simulink library "srx_platform"  (Simulink 8.2)
settings: Solver=ode1  StartTime=0.0  StopTime=Inf  FixedStep=0.001  RelTol=1e-3
PostLoadFcn:
  | , if any(exist('dsrtsu_mdlpostloadfcn', 'file') == [2, 3, 6]), try dsrtsu_mdlpostloadfcn('Execute', bdroot); catch fprintf('Error in PostLoadFcn (dsrtsu_mdlpostloadfcn) for model "%s":\n %s\n', bdroot, lasterr); end, end,
libraries: rtican x23, rtiethernetudplib x4, srx_initialize x4, rtiflashlib x2, topr5_adapter x1
(part 1 of 6)
settings Model: DSRTSU_INTERNAL_RTI_VER=450  DSRTSU_INTERNAL_RTI_TYPE=rti1401  DSRTSU_INTERNAL_RTIFPGA=40  Creator=leidos  LastModifiedBy=rushk1

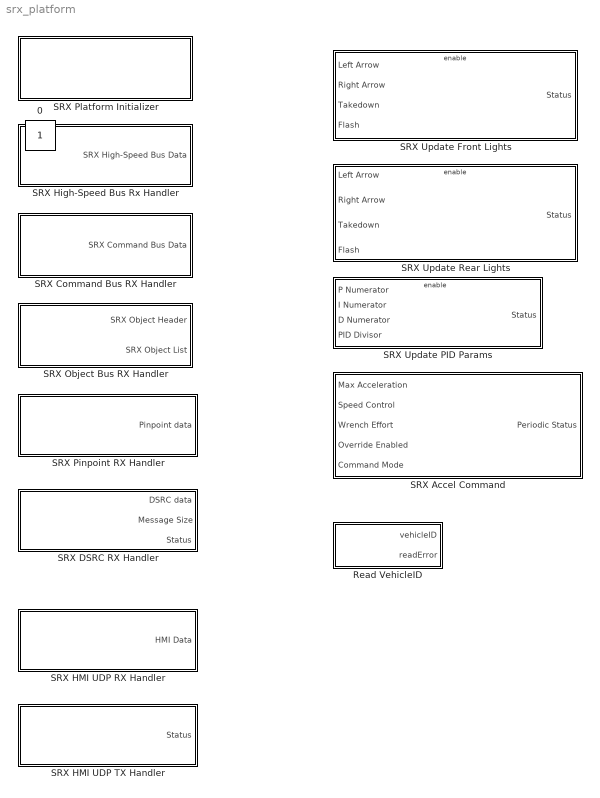
== system srx_platform ==
  Read VehicleID : Subsystem
  SRX Accel Command : Subsystem
  SRX Command Bus RX Handler : Subsystem
  SRX DSRC RX Handler : Subsystem
  SRX HMI UDP RX Handler : Subsystem
  SRX HMI UDP TX Handler : Subsystem
  SRX High-Speed Bus Rx Handler : Subsystem
  SRX Object Bus RX Handler : Subsystem
  SRX Pinpoint RX Handler : Subsystem
  SRX Platform Initializer : Subsystem  mask(SRX Platform Initializer){enable_can1=on, enable_can2=on, enable_can3=on, enable_can4=off}
      mask help:
      | This block contains setup blocks for all the platform devices on the
      | current SRX platform and maps physical devices to virutal ones.  This
      | include 4 CAN busses and 2 UDP Ports.
      |
      | For UDP, the curret configuration is:
      |
      | Autobox IP Address: 192.168.88.20
      | Linux PC IP Address:192.168.88.10
      |
      | Pinpoint Rx Port: 5000
      | DSRC Tx/Rx Port: 5001
      | Test interface TX/RX Port: 5002
      mask init:
      | can1_block = find_system(gcb,'LookUnderMasks', 'on',...
      |     'FollowLinks', 'on', 'Name', 'Can1Init');
      | can2_block = find_system(gcb,'LookUnderMasks', 'on',...
      |     'FollowLinks', 'on', 'Name', 'Can2Init');
      | can3_block = find_system(gcb,'LookUnderMasks', 'on',...
      |     'FollowLinks', 'on', 'Name', 'Can3Init');
      | can4_block = find_system(gcb,'LookUnderMasks', 'on',...
      |     'FollowLinks', 'on', 'Name', 'Can4Init');
      | 
      | if enable_can1
      |     if isempty(can1_block)
      |         add_block('srx_initialize/SRX High-Speed Bus Initializer',...
      |             [gcb,'/Can1Init']);
      |     end
      | else 
      |     if ~isempty(can1_block)
      |         delete_block(can1_block);
      |     end 
      | end
      | 
      | if enable_can2
      |     if isempty(can2_block)
      |         add_block('srx_initialize/SRX Object Bus Initializer',...
      |             [gcb,'/Can2Init']);
      |     end
      | else 
      |     if ~isempty(can2_block)
      |         delete_block(can2_block);
      |     end 
      | end
      | 
      | if enable_can3
      |     if isempty(can3_block)
      |         add_block('srx_initialize/SRX Command Bus Initializer',...
      |             [gcb,'/Can3Init']);
      |     end
      | else 
      |     if ~isempty(can3_block)
      |         delete_block(can3_block);
      |     end 
      | end
      | 
      | if enable_can4
      |     if isempty(can4_block)
      |         add_block('srx_initialize/SRX Logging Bus Initializer',...
      |             [gcb,'/Can4Init']);
      |     end
      | else 
      |     if ~isempty(can4_block)
      |         delete_block(can4_block);
      |     end 
      | end
      mask DialogControl Control2 Prompt: Initialize SRX High-Speed Bus:
      mask DialogControl Control3 Prompt: Initialize SRX Object Bus:
      mask DialogControl Control4 Prompt: Initialize SRX Command Bus:
      mask DialogControl Control5 Prompt: Initialize SRX Logging Bus:
  SRX Update Front Lights : Subsystem  TreatAsAtomicUnit=on
  SRX Update PID Params : Subsystem
  SRX Update Rear Lights : Subsystem  TreatAsAtomicUnit=on
  0 : Constant  IOType=siggen

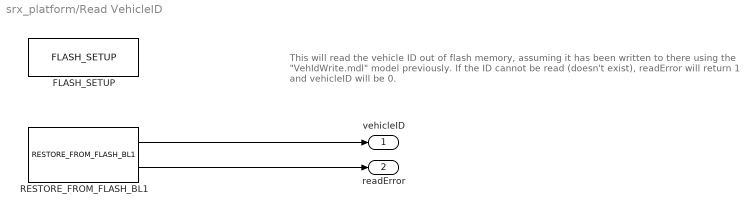
== system srx_platform/Read VehicleID ==
  note: This will read the vehicle ID out of flash memory,
      | assuming it has been written to there using the "VehIdWrite.mdl" model
      | previously. If the ID cannot be read (doesn't exist), readError will return 1 and vehicleID will be 0.
  FLASH_SETUP : rtiflashlib/FLASH_SETUP  UseNVRAM=on  UseFlrec=off  UseRestForFlRec=on  FlRecMemSize=13  BufferOverrunMode=Discard new data  TLCFileName=rtiflashsetup  Reserved1=[]  Reserved2=[]  Reserved3=[]  Reserved4=[]  DSProperties=struct('RTI',struct('Version',uint32(1),'BlockType',struct('isSLSource',uint8(0),'isSLSink',uint8(0),'isHWSource',uint8(0),'isHWSink',uint8(0),'isSetup',uint8(1),'isInline',uint8(1),'isNonInline',uint8(0),'isInterrupt',uint8(0),'isChannelwise',uint8(0)),'IOBoardType','DSFLASH','UnitType','FLASH','Identifier','SETUP','DialogType','SL','BlockSet','NONE','SlaveProcessor','NONE'))  RTIBlockInterface=struct('OutputPortsActive',0,'OutputPortsWidth',int32(0),'BlockDisplay',{{'Flash\nSetup','center'}},'IconTransparency','off','InitLevel',3,'BlockName',struct('Token',{{'FLASH_SETUP'}}),'MaskDescription',['Initializes the flash memory for flight recorder and non-volatile data interface blocks.'])  RTIBlockParameters=struct('UseNVRAM',{{logical(1),'ON',[0 1]}},'UseFlrec',{{logical(0),'ON',[0 1]}},'UseRestForFlRec',{{logical(1),'ON',[0 1]}},'FlRecMemSize',{{13,'OFF',[]}},'BufferOverrunMode',{{1,'OFF',[1 2]}},'TLCFileName',{{'rtiflashsetup','OFF',[]}})  RTISFcnParameters=struct('UseNVRAM','double','UseFlrec','double','UseRestForFlRec','double','FlRecMemSize','double','BufferOverrunMode','double','TLCFileName','char')  RTIBlockParaDefault=struct('UseNVRAM',0,'UseFlrec',1,'UseRestForFlRec',1,'FlRecMemSize',13,'BufferOverrunMode',1,'TLCFileName','rtiflashsetup')
  RESTORE_FROM_FLASH_BL1 : rtiflashlib/RESTORE_FROM_FLASH_BL1  DataLabel=vehID  NumOfElements=1  DataType=UInt8  DefaultValues=0  TLCFileName=rtinvdatarestore  Reserved1=[]  Reserved2=[]  Reserved3=[]  Reserved4=[]  DSProperties=struct('RTI',struct('Version',uint32(1),'BlockType',struct('isSLSource',uint8(1),'isSLSink',uint8(0),'isHWSource',uint8(0),'isHWSink',uint8(0),'isSetup',uint8(0),'isInline',uint8(1),'isNonInline',uint8(0),'isInterrupt',uint8(0),'isChannelwise',uint8(0)),'IOBoardType','DSFLASH','UnitType','FLASH','Identifier','NVDATARESTORE','DialogType','SL','BlockSet','NONE','SlaveProcessor','NONE'))  RTIBlockInterface=struct('OutputPortsActive',[1 1],'OutputPortsWidth',int32([1 1]),'OutputPortsName',{{'vehID','Status'}},'OutputPortsDataType',{{'SS_UINT8','SS_UINT16'}},'IconTransparency','on','InitLevel',3,'BlockName',struct('Token',{{'RESTORE_FROM_FLASH_BL1'}}),'MaskDescription',['To restore data from non-volatile flash memory'])  RTIBlockParameters=struct('DataLabel',{{'vehID','OFF',[]}},'NumOfElements',{{1,'ON',[1 inf]}},'DataType',{{8,'OFF',[]}},'DefaultValues',{{0,'OFF',[]}},'TLCFileName',{{'rtinvdatarestore','OFF',[]}})  RTISFcnParameters=struct('DataLabel','char','NumOfElements','double','DataType','double','DefaultValues','double','TLCFileName','char')  RTIBlockParaDefault=struct('DataLabel','Data','NumOfElements',1,'DataType',1,'DefaultValues',0,'TLCFileName','rtinvdatarestore')
  vehicleID : Outport
  readError : Outport  Port=2
  wires:
  RESTORE_FROM_FLASH_BL1/1 -> vehicleID/1
  RESTORE_FROM_FLASH_BL1/2 -> readError/1

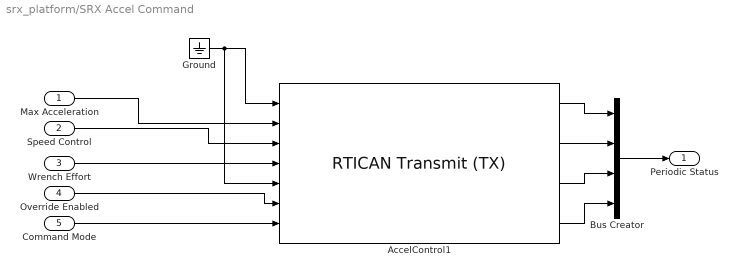
== system srx_platform/SRX Accel Command ==
  Max Acceleration : Inport
  Speed Control : Inport  Port=2
  Wrench Effort : Inport  Port=3
  Override Enabled : Inport  Port=4
  Command Mode : Inport  Port=5
  AccelControl1 : rtican/RTICAN Transmit (TX)   Reserved1=[]  Reserved2=[]  Reserved3=[]  Reserved4=[]  SfcnMessage=[]  Msg_Struct=[]  BoardTypeNo=[]  BoardNo=[]  ChannelNo=[]  Parameters=[]  DialogFcn=[]  UnitName=[]  Revision=[]  UnitValues=[]  DSProperties=struct('RTI',struct('Version',uint32(5),'BlockType',struct('isSLSource',uint8(1),'isSLSink',uint8(1),'isHWSource',uint8(0),'isHWSink',uint8(0),'isSetup',uint8(0),'isInline',uint8(1),'isNonInline',uint8(0),'isInterrupt',uint8(0),'isChannelwise',uint8(0)),'IOBoardType','RTICAN','UnitType','MESSAGE','Identifier','TX','DialogType','MSVC','BlockSet','RTICAN','SlaveProcessor','CAN'))  RTIBlockInterface=struct('InputPortsWidth',int32([1 1 1 1 1 1 1]),'InputPortsActive',[1 1 1 1 1 1 1],'InputPortsName',{{'Checksum','MaxAccel','SpeedControl','WrenchEffort','CommandCntr','OverrideEnable','CommandMode'}},'InputPortsDataType',{{'SS_UINT8','SS_DOUBLE','SS_DOUBLE','SS_DOUBLE','SS_UINT8','SS_BOOLEAN','SS_UINT8'}},'OutputPortsWidth',int32([1 1 1 1]),'OutputPortsActive',[1 1 1 1],'OutputPortsName',{{['TX status'],['TX time'],['TX delta time'],['TX delay time']}},'DialogFcn','rtican_message_interface_gui','BlockDisplay',{{'','center'}},'IconTransparency','on','InitLevel',3,'BlockName',struct('Token',{{'AccelControl'}}),'SampleTime',{{-1}},'TriggerPort',{{'none'}},'EnablePort',{{'none'}})  RTIBlockParameters=struct('BoardTypeNo',{{1,'OFF',[]}},'BoardNo',{{2,'ON',[1 16]}},'ChannelNo',{{1,'ON',[1 2]}},'Parameters',{{struct('DataFileSupport',struct('DataFileSelectedMaster',1,'DataFileSelectedLocal',1,'DataFileName','c:\users\leidos\development\carmaplatform\microautobox\src\data_files\srx_command.dbc|','DataFileDate',['17-Aug-2015 10:52:13'],'SelectedFile','..\data_files\srx_command.dbc','InterfaceFcn','rtican_dbc_file_parser'),'Options',struct('StatusSelected',1,'TimeSelected',1,'DeltaTimeSelected',1,'DelayTimeSelected',1,'DelayTimeTXCommandSelected',0,'EncodeSetUnusedBitsToOne',0,'EnableMsgLoopback',0,'TriggerPort',struct('Selected',0,'TriggerType',0),'EnablePortSelected',0,'SignalOnPortnameSelected',1,'UserCoding',struct('Selected',1,'InterfaceFile','UserEncodingFile','FcnName','AccelCommandEncode','InportSelected',0,'InportWidth',1,'OutportSelected',0,'OutportWidth',1),'TerminationMsg',struct('Selected',0,'Byte0_7','0'),'InitialMsg',struct('Selected',0,'Byte0_7','0')),'Message',struct('MsgOnBlocknameSelected',1,'MsgName','AccelControl','MsgIdFormat',0,'MsgId',256,'MsgLength',8,'NumSignals',7,'SampleTime',-1,'StartTime',struct('Selected',0,'Value',0),'AutoRepeatTime',struct('Selected',1,'Value',0.02),'Timeout',struct('Selected',1,'Value',0.2),'DelayTime',struct('Selected',0,'Value',0.1),'Signal',struct('SgnName',{'Checksum','MaxAccel','SpeedControl','WrenchEffort','CommandCntr','OverrideEnable','CommandMode'},'SgnStartBit',{0,8,24,40,56,58,59},'SgnLength',{8,16,16,16,2,1,2},'SgnType',{0,0,0,0,0,0,0},'ModeValue',{-1,-1,-1,-1,-1,-1,-1},'DataType',{0,0,0,0,0,0,0},'ByteLayout',{2,2,2,2,2,2,2},'Factor',{1,0.03125,0.03125,0.025,1,1,1},'Offset',{0,0,0,-100,0,0,0},'SgnComment',{{''},{''},{''},{''},{''},{''},{''}},'SgnUnit',{'','(km/h)/s','km/h','%','','',''},'Min',{0,0,0,0,0,0,0},'Max',{0,0,0,0,0,0,0},'SLDataType',{'SS_UINT8','SS_DOUBLE','SS_DOUBLE','SS_DOUBLE','SS_UINT8','SS_BOOLEAN','SS_UINT8'}),'MsgIdNumFormat',0,'MsgComment',{{''}}),'Version',1.2,'general',struct('isFromLib',0)),'OFF',[]}},'GroupId',{{struct('Group',{{'RTICAN'}},'No',3,'Behavior',{{'NAMECHANGE'}},'BlockType',{{'SINK'}},'NameChangeFlag',0),'OFF',[]}},'SFcnRTICANMessage',{{struct('MsgType','TX','SFcnPortType','Scalar','MsgName','AccelControl','MsgIdFormat','STD','MsgId',256,'MsgLength',8,'NumSignals',7,'SampleTime',-1,'StartTime',struct('Selected','no','Value',0),'AutoRepeatTime',struct('Selected','yes','Value',0.02),'Timeout',struct('Selected','yes','Value',0.2),'Signal',struct('SgnName',{'Checksum','MaxAccel','SpeedControl','WrenchEffort','CommandCntr','OverrideEnable','CommandMode'},'SgnStartBit',{0,8,24,40,56,58,59},'SgnLength',{8,16,16,16,2,1,2},'SgnType',{'standard','standard','standard','standard','standard','standard','standard'},'ModeValue',{-1,-1,-1,-1,-1,-1,-1},'DataType',{['unsigned int'],['unsigned int'],['unsigned int'],['unsigned int'],['unsigned int'],['unsigned int'],['unsigned int']},'ByteLayout',{['motorola back.'],['motorola back.'],['motorola back.'],['motorola back.'],['motorola back.'],['motorola back.'],['motorola back.']},'Factor',{1,0.03125,0.03125,0.025,1,1,1},'Offset',{0,0,0,-100,0,0,0},'SLDataType',{'SS_UINT8','SS_DOUBLE','SS_DOUBLE','SS_DOUBLE','SS_UINT8','SS_BOOLEAN','SS_UINT8'}),'StatusSelected','yes','TimeSelected','yes','DeltaTimeSelected','yes','DelayTimeSelected','yes','DelayTimeTXCommandSelected','no','EncodeSetUnusedBitsToOne','no','EnableMsgLoopback','no','TriggerPort',struct('Selected','no','TriggerType',0),'EnablePortSelected','no','UserCoding',struct('Selected','yes','InterfaceFile','UserEncodingFile','FcnName','AccelCommandEncode','InportSelected','no','InportWidth',1,'OutportSelected','no','OutportWidth',1),'TerminationMsg',struct('Selected','no','Byte0','0x00','Byte1','0x00','Byte2','0x00','Byte3','0x00','Byte4','0x00','Byte5','0x00','Byte6','0x00','Byte7','0x00'),'InitialMsg',struct('Selected','no','Byte0','0x00','Byte1','0x00','Byte2','0x00','Byte3','0x00','Byte4','0x00','Byte5','0x00','Byte6','0x00','Byte7','0x00'),'BoardType','DS1','BoardNo',2,'ControllerNo',1),'OFF',[]}},'TLCFileName',{{'rtican_tx_message','OFF',[]}})  RTISFcnParameters=struct('SFcnRTICANMessage','struct','TLCFileName','char')  RTIBlockParaDefault=struct('BoardTypeNo',4302,'BoardNo',1,'ChannelNo',1,'Parameters',struct('DataFileSupport',struct('DataFileSelectedMaster',0,'DataFileSelectedLocal',0,'DataFileName','','DataFileDate','','SelectedFile',['<no file selected>']),'Options',struct('StatusSelected',1,'TimeSelected',1,'DeltaTimeSelected',1,'DelayTimeSelected',1,'DelayTimeTXCommandSelected',0,'EncodeSetUnusedBitsToOne',0,'EnableMsgLoopback',0,'TriggerPort',struct('Selected',0,'TriggerType','rising'),'EnablePortSelected',0,'SignalOnPortnameSelected',1,'UserCoding',struct('Selected',0,'InterfaceFile','UserEncodingFile','FcnName','UserEncodeFcn','InportSelected',0,'InportWidth',1,'OutportSelected',0,'OutportWidth',1),'TerminationMsg',struct('Selected',0,'Byte0_7','0'),'InitialMsg',struct('Selected',0,'Byte0_7','0')),'Message',struct('MsgOnBlocknameSelected',0,'MsgName',['TX Message'],'MsgIdFormat',0,'MsgId',100,'MsgLength',8,'NumSignals',1,'SampleTime',-1,'StartTime',struct('Selected',0,'Value',0),'AutoRepeatTime',struct('Selected',0,'Value',0.1),'Timeout',struct('Selected',0,'Value',0.1),'DelayTime',struct('Selected',0,'Value',0.1),'Signal',struct('SgnName',['TX signal'],'SgnStartBit',0,'SgnLength',8,'SgnType',0,'ModeValue',-1,'DataType',0,'SLDataType','SS_DOUBLE','ByteLayout',0,'Factor',1,'Offset',0,'Min',0,'Max',255,'SgnComment',{{}},'SgnUnit',''),'MsgIdNumFormat',0,'MsgComment',{{''}}),'Version',1.2,'general',struct('isFromLib',1)),'GroupId',struct('Group',{{'RTICAN'}},'No',1,'Behavior',{{'NAMECHANGE'}},'BlockType',{{'SINK'}},'NameChangeFlag',0),'SFcnRTICANMessage',struct('MsgType','TX','MsgName',['TX Message'],'MsgIdFormat','STD','MsgId',100,'MsgLength',2,'NumSignals',1,'SampleTime',-1,'StartTime',struct('Selected','no','Value',0),'AutoRepeatTime',struct('Selected','no','Value',0.1),'Timeout',struct('Selected','no','Value',0.1),'DelayTime',struct('Selected','no','Value',0.1),'Signal',struct('SgnName',['TX signal'],'SgnStartBit',0,'SgnLength',8,'SgnType','standard','ModeValue',-1,'DataType',['unsigned int'],'ByteLayout',['little endian'],'SLDataType','SS_DOUBLE','Factor',1,'Offset',0),'StatusSelected','yes','TimeSelected','yes','DeltaTimeSelected','yes','DelayTimeSelected','yes','EnablePortSelected','no','EnableMsgLoopback','no','DelayTimeTXCommandSelected','no','EncodeSetUnusedBitsToOne','no','UserCoding',struct('Selected','no','InterfaceFile','UserDecodingFile','FcnName','UserDecodeFcn','InportSelected','no','InportWidth',1,'OutportSelected','no','OutportWidth',1),'TerminationMsg',struct('Selected','no','Byte0','0x00','Byte1','0x00','Byte2','0x00','Byte3','0x00','Byte4','0x00','Byte5','0x00','Byte6','0x00','Byte7','0x00'),'InitialMsg',struct('Selected','no','Byte0','0x00','Byte1','0x00','Byte2','0x00','Byte3','0x00','Byte4','0x00','Byte5','0x00','Byte6','0x00','Byte7','0x00'),'TriggerPort',struct('Selected','no','TriggerType','rising'),'BoardType','DS4302','BoardNo',1,'ControllerNo',1,'SFcnPortType','Scalar'),'TLCFileName','rtican_tx_message')
      settings: AttributesFormatString=Group Id: RTICAN3\n
  Bus Creator : BusCreator
  Ground : Ground
  Periodic Status : Outport
  wires:
  Max Acceleration/1 -> AccelControl1/2
  Wrench Effort/1 -> AccelControl1/4
  Speed Control/1 -> AccelControl1/3
  Override Enabled/1 -> AccelControl1/6
  Command Mode/1 -> AccelControl1/7
  AccelControl1/2 -> Bus Creator/2
  AccelControl1/1 -> Bus Creator/1
  AccelControl1/3 -> Bus Creator/3
  AccelControl1/4 -> Bus Creator/4
  Bus Creator/1 -> Periodic Status/1
  Ground/1 -> AccelControl1/5, AccelControl1/1
